simulink model "Inter_story_damped_structure_MFD_LSTM"  (R2024a)
settings: Solver=ode4  StartTime=0.0  StopTime=tend  FixedStep=dt  RelTol=1e-3
values from neighbouring files (symbols this model uses):
  A0 = 0.4    [Base_isolated_structure_main.m]    (also in Inter_story_damped_structure_MBW_main.m = [zeros(Ns) eye(Ns);-M\K -M\C]; Inter_story_damped_structure_MFD_main.m = [zeros(Ns) eye(Ns);-M\K -M\C])
  B1 = [zeros(Ns,1+Ns);-ones(Ns,1) -M\Re]    [Inter_story_damped_structure_MBW_main.m]    (also in Inter_story_damped_structure_MFD_main.m)
  C0 = eye(2*Ns)    [Inter_story_damped_structure_MBW_main.m]    (also in Inter_story_damped_structure_MFD_main.m)
  D1 = zeros(2*Ns,1+Ns)    [Inter_story_damped_structure_MBW_main.m]    (also in Inter_story_damped_structure_MFD_main.m)
  dt = 0.002    [BLWN_training_data_prep.m]    (also in Base_isolated_structure_main.m; Inter_story_damped_structure_MBW_main.m; Inter_story_damped_structure_MFD_main.m)
  Ns = 5    [Inter_story_damped_structure_MBW_main.m]    (also in Inter_story_damped_structure_MFD_main.m)
libraries: deeplib x1
settings Model: Creator=hongwei  LastModifiedBy=li292
settings DataIOCC: SaveTime=off  ReturnWorkspaceOutputs=off
settings OptimizationCC: ReuseModelBlockBuffer=off
settings DebuggingCC: SigSpecEnsureSampleTimeMsg=none
settings RTWCC: GPUComputeCapability=3.5

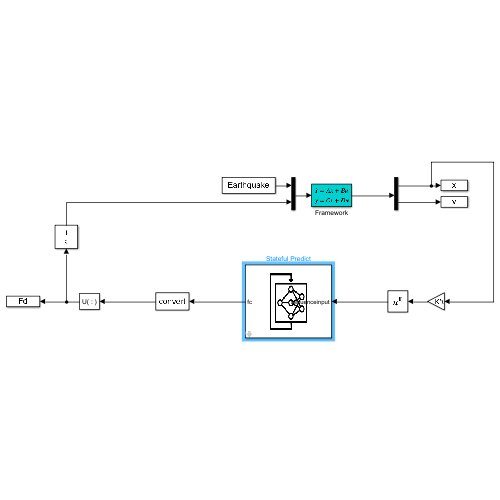
[thumbnail: Simulink's stored preview of the top-level diagram]
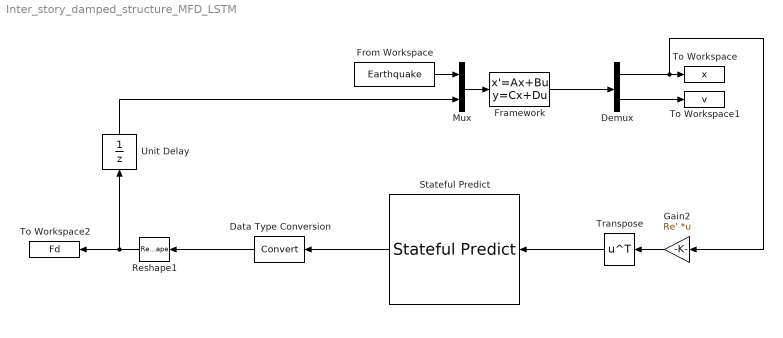
== system Inter_story_damped_structure_MFD_LSTM ==
  Data Type Conversion : DataTypeConversion  SaturateOnIntegerOverflow=off  RndMeth=Floor
  Demux : Demux  Outputs=2
  Framework : StateSpace  A=A0  B=B1  C=C0  D=D1  InitialCondition=zeros(2*Ns,1)
  From Workspace : FromWorkspace  VariableName=Earthquake  SampleTime=dt
  Gain2 : Gain  Gain=Re'  Multiplication=Matrix(K*u)
  Mux : Mux  Inputs=2
  Reshape1 : Reshape
  Stateful Predict : deeplib/Stateful Predict  Network=Network from MAT-file  NetworkFunction=untitled  NetworkFilePath=MFD_Simulink.mat  InputDataFormats={ 'sequenceinput', 'TBC' }  SampleTime=dt  ForceInterpretedSim=off  EnableDLNetwork=on  LastKnownNetworkFilePath=''  LastKnownNetworkTimeStamp=''
  To Workspace : ToWorkspace  VariableName=x  SampleTime=-1
  To Workspace1 : ToWorkspace  VariableName=v  SampleTime=-1
  To Workspace2 : ToWorkspace  VariableName=Fd  SampleTime=-1
  Transpose : Math  Operator=transpose
  Unit Delay : UnitDelay  InitialCondition=zeros(5,1)  SampleTime=-1  HasFrameUpgradeWarning=on
  wires:
  Framework/1 -> Demux/1
  Demux/1 -> To Workspace/1, Gain2/1
  Demux/2 -> To Workspace1/1
  Mux/1 -> Framework/1
  From Workspace/1 -> Mux/1
  Transpose/1 -> Stateful Predict/1
  Stateful Predict/1 -> Data Type Conversion/1
  Data Type Conversion/1 -> Reshape1/1
  Gain2/1 -> Transpose/1
  Reshape1/1 -> Unit Delay/1, To Workspace2/1
  Unit Delay/1 -> Mux/2
